simulink model "lab6_1"  (R2018b)
settings: Solver=VariableStepAuto  StartTime=0.0  StopTime=10.0  RelTol=1e-3
libraries: hdlsllib x8
settings Model: Creator=mllax8  LastModifiedBy=mllax8

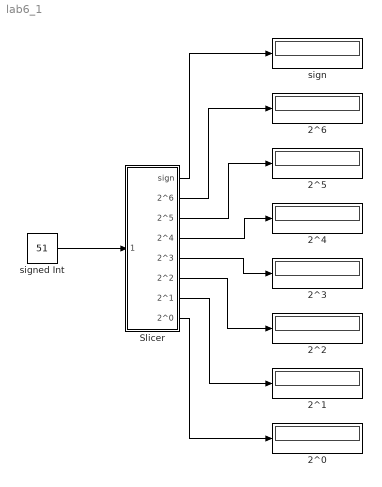
== system lab6_1 ==
  2^{0..6} (7 alike) : Display
  Slicer : Subsystem
  sign : Display
  signed Int : Constant  Value=51  OutDataTypeStr=int8
  wires:
  signed Int/1 -> Slicer/1(sign Int)
  Slicer/8("2^0 ") -> 2^0/1
  Slicer/7(2^1) -> 2^1/1
  Slicer/6(2^2) -> 2^2/1
  Slicer/1(sign) -> sign/1
  Slicer/2(2^6) -> 2^6/1
  Slicer/3(2^5) -> 2^5/1
  Slicer/4(2^4) -> 2^4/1
  Slicer/5(2^3) -> 2^3/1

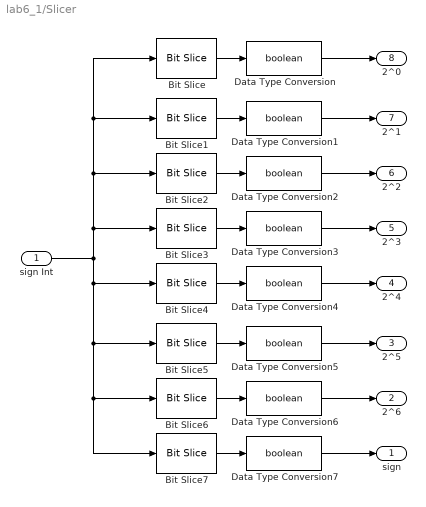
== system lab6_1/Slicer ==
  sign Int : Inport  OutDataTypeStr=int8  SampleTime=1
  Bit Slice : hdlsllib/Logic and Bit Operations/Bit Slice  lidx=0  ridx=0
  Bit Slice1 : hdlsllib/Logic and Bit Operations/Bit Slice  lidx=1  ridx=1
  Bit Slice2 : hdlsllib/Logic and Bit Operations/Bit Slice  lidx=2  ridx=2
  Bit Slice3 : hdlsllib/Logic and Bit Operations/Bit Slice  lidx=3  ridx=3
  Bit Slice4 : hdlsllib/Logic and Bit Operations/Bit Slice  lidx=4  ridx=4
  Bit Slice5 : hdlsllib/Logic and Bit Operations/Bit Slice  lidx=5  ridx=5
  Bit Slice6 : hdlsllib/Logic and Bit Operations/Bit Slice  lidx=6  ridx=6
  Bit Slice7 : hdlsllib/Logic and Bit Operations/Bit Slice  lidx=7  ridx=7
  Data Type Conversion{,1..7} (8 alike) : DataTypeConversion  OutDataTypeStr=boolean
  sign : Outport
  2^6 : Outport  Port=2
  2^5 : Outport  Port=3
  2^4 : Outport  Port=4
  2^3 : Outport  Port=5
  2^2 : Outport  Port=6
  2^1 : Outport  Port=7
  "2^0 " : Outport  Port=8
  wires:
  Data Type Conversion/1 -> "2^0 "/1
  Data Type Conversion5/1 -> 2^5/1
  Bit Slice1/1 -> Data Type Conversion1/1
  Bit Slice5/1 -> Data Type Conversion5/1
  Bit Slice7/1 -> Data Type Conversion7/1
  Bit Slice2/1 -> Data Type Conversion2/1
  Bit Slice3/1 -> Data Type Conversion3/1
  Data Type Conversion6/1 -> 2^6/1
  Bit Slice4/1 -> Data Type Conversion4/1
  sign Int/1 -> Bit Slice4/1, Bit Slice5/1, Bit Slice6/1, Bit Slice7/1, Bit Slice3/1, Bit Slice2/1, Bit Slice1/1, Bit Slice/1
  Data Type Conversion1/1 -> 2^1/1
  Data Type Conversion2/1 -> 2^2/1
  Bit Slice/1 -> Data Type Conversion/1
  Bit Slice6/1 -> Data Type Conversion6/1
  Data Type Conversion3/1 -> 2^3/1
  Data Type Conversion4/1 -> 2^4/1
  Data Type Conversion7/1 -> sign/1
